simulink model "adaptive_PID"  (R2024a)
settings: Solver=FixedStepAuto  StartTime=0.0  StopTime=50  FixedStep=dt  RelTol=1e-3
undefined symbols (not defined in the file): DiscIntNeverNeededParam
libraries: simulink x1
settings Model: Creator=User  LastModifiedBy=Bocchio
settings DebuggingCC: UnconnectedInputMsg=warning  UnconnectedOutputMsg=warning  UnconnectedLineMsg=warning
settings ModelReferenceCC: EnableRefExpFcnMdlSchedulingChecks=on
settings RTWCC: GPUComputeCapability=3.5  DLArmComputeVersion=19.05

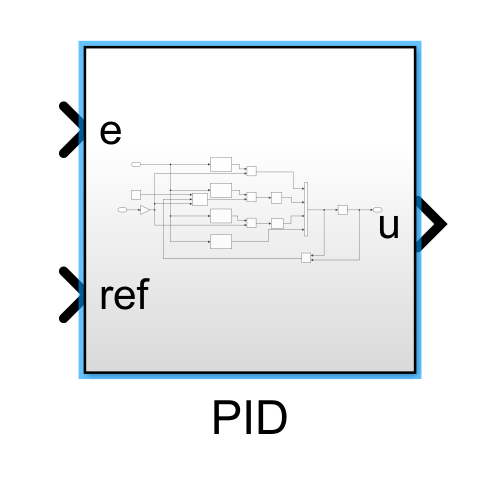
[thumbnail: Simulink's stored preview of the top-level diagram]
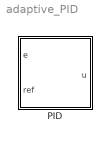
== system adaptive_PID ==
  PID : Subsystem

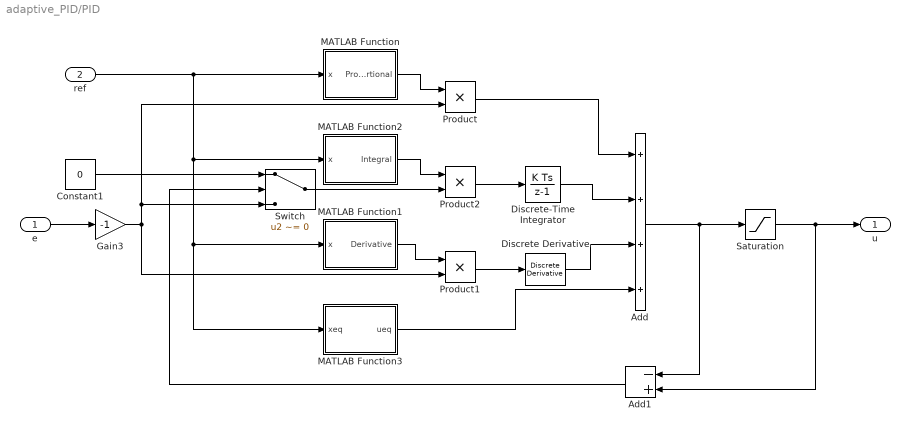
== system adaptive_PID/PID ==
  e : Inport
  ref : Inport  Port=2
  Add : Sum  Inputs=++++
  Add1 : Sum  Inputs=-+
  Constant1 : Constant  Value=0
  Discrete Derivative : simulink/Discrete/Discrete Derivative  gainval=1.0  ICPrevScaledInput=0.0  OutMin=[]  OutMax=[]  OutDataType=fixdt(1, 16)  OutScaling=2^-10  DoSatur=off
  Discrete-Time Integrator : DiscreteIntegrator  SampleTime=-1  ICPrevOutput=DiscIntNeverNeededParam  ICPrevScaledInput=DiscIntNeverNeededParam
  Gain3 : Gain  Gain=-1
  MATLAB Function : MATLAB Function  TreatAsAtomicUnit=on
  MATLAB Function1 : MATLAB Function  TreatAsAtomicUnit=on
  MATLAB Function2 : MATLAB Function  TreatAsAtomicUnit=on
  MATLAB Function3 : MATLAB Function  TreatAsAtomicUnit=on
  Product : Product
  Product1 : Product
  Product2 : Product
  Saturation : Saturate  UpperLimit=1  LowerLimit=0
  Switch : Switch  Criteria=u2 ~= 0  SaturateOnIntegerOverflow=off  InputSameDT=off
  u : Outport
  wires:
  MATLAB Function3/1(ueq) -> Add/4
  e/1 -> Gain3/1
  Saturation/1 -> u/1, Add1/2
  Add/1 -> Saturation/1, Add1/1
  Constant1/1 -> Switch/1
  Add1/1 -> Switch/2
  Gain3/1 -> Switch/3, Product/2, Product1/2
  Product/1 -> Add/1
  MATLAB Function/1(Proportional) -> Product/1
  Product1/1 -> Discrete Derivative/1
  MATLAB Function1/1(Derivative) -> Product1/1
  Product2/1 -> Discrete-Time Integrator/1
  MATLAB Function2/1(Integral) -> Product2/1
  Switch/1 -> Product2/2
  ref/1 -> MATLAB Function3/1(xeq), MATLAB Function1/1(x), MATLAB Function2/1(x), MATLAB Function/1(x)
  Discrete-Time Integrator/1 -> Add/2
  Discrete Derivative/1 -> Add/3

== matlab function adaptive_PID/PID/MATLAB Function1 ==
  data: x input; Derivative output
function Derivative = Derivative(x)

vect_pos=0.0005:0.0005:0.0185;
Kd=[-3.13284561278702	-3.15696834297852	-3.55596908354099	-4.07211547270984	-4.52885655579409	-5.03467071847558	-5.67368160958219	-6.13040622703350	-6.65900086248431	-7.20427821963870	-7.79296644491808	-8.26092294070224	-8.91573932517159	-9.51445223185005	-10.0073933096390	-10.5915963054668	-11.1707021043877	-11.7514268462752	-12.2320444397896	-12.8718043152667	-13.5079237552714	-14.0081015881516	-14.6774203594397	-15.2753544831799	-15.7810311815792	-16.5628549756766	-17.4462648456270	-18.5186925601413	-19.1642011529234	-19.8229727022934	-20.6805255599888	-21.4746229693166	-22.5687040270238	-23.8586191312697	-26.1242011711683	-28.3053228476865	-31.1934330156860];

if x<=vect_pos(1)
    Derivative=Kd(1);
elseif x>=vect_pos(1) && x<=vect_pos(end)
    Derivative=interp1(vect_pos,Kd,x);
else 
    Derivative=Kd(end);
end

== matlab function adaptive_PID/PID/MATLAB Function2 ==
  data: x input; Integral output
function Integral = Integral(x)

vect_pos=0.0005:0.0005:0.0185;
Ki=[-21.5916724653951	-21.7579270957351	-24.5078529996838	-28.0651504718742	-31.2130246688002	-34.6991121045807	-39.1031956656343	-42.2509563808898	-45.8940475657967	-49.6521166038685	-53.7093747376836	-56.9345459187291	-61.4475614470809	-65.5739100066915	-68.9712757284227	-72.9976215169708	-76.9888372609179	-80.9912108117267	-84.3036426844985	-88.7128882698608	-93.0970438571618	-96.5442855271381	-101.157251970683	-105.278233133299	-108.763373160837	-114.151727830759	-120.240216994353	-127.631423206396	-132.080289135844	-136.620563787574	-142.530845593210	-148.003790413038	-155.544232161009	-164.434368440105	-180.048832539233	-195.081193104444	-214.986141033221];

if x<=vect_pos(1)
    Integral=Ki(1);
elseif x>=vect_pos(1) && x<=vect_pos(end)
    Integral=interp1(vect_pos,Ki,x);
else 
    Integral=Ki(end);
end

== matlab function adaptive_PID/PID/MATLAB Function3 ==
  data: xeq input; ueq output
function ueq = ueq(xeq)
BallMass=0.0620;
g=9.81;
m=11.3044;
Res=4;
Kem_1=[6.72059206644115e-05	6.92145376989519e-05	6.92332150285897e-05	6.80659146785482e-05	6.99479714473845e-05	7.05722629122651e-05	6.80128124860478e-05	7.01221702001213e-05	7.05016878442255e-05	7.05515419323440e-05	6.98455307642310e-05	7.13055533313152e-05	6.96274521174565e-05	6.90147402074580e-05	6.99419931300404e-05	6.95805738707539e-05	6.93269258852514e-05	6.90843621353604e-05	7.00006512636940e-05	6.91149414076029e-05	6.97519014539535e-05	6.83573053782350e-05	6.89933518537361e-05	6.79953062557338e-05	6.77206336827605e-05	6.82595333358458e-05	6.6494e-05	6.41548968339966e-05	6.08172215535155e-05	6.05299131311581e-05	6.01818568879911e-05	5.87123846492744e-05	5.77159494392489e-05	5.52986546480238e-05	5.22809928128838e-05	4.60062308129917e-05	4.12885327629886e-05	3.57707157204477e-05	2.88156521526937e-05	2.23928764595895e-05	1.69237291476886e-05];
if xeq>=0.0185
    K1f=Kem_1(1);
    ieq = sqrt((BallMass*g)/K1f)*xeq;
    ueq = (Res*ieq)/m;
elseif xeq<0.0185 && xeq>0
    K1f = Kem_1(round(xeq*length(Kem_1)/0.02));
    ieq = sqrt((BallMass*g)/K1f)*xeq;
    ueq = (Res*ieq)/m;
else 
    K1f=Kem_1(end);
    ieq = sqrt((BallMass*g)/K1f)*xeq;
    ueq = (Res*ieq)/m;

== matlab function adaptive_PID/PID/MATLAB Function ==
  data: x input; Proportional output
function Proportional = Proportional(x)

vect_pos=0.0005:0.0005:0.0185;
Kp=[-16.4491186822817	-16.5757759456467	-18.6707436992577	-21.3807888984900	-23.7789243993465	-26.4347198714141	-29.7898695615811	-32.1879186090389	-34.9633237735508	-37.8263221689982	-40.9172508904643	-43.3742733194918	-46.8124103216076	-49.9559739936797	-52.5441788700475	-55.6115577327956	-58.6521735796689	-61.7012897448753	-64.2247897233749	-67.5838719829448	-70.9238400049996	-73.5500417245203	-77.0643240307596	-80.2037986749755	-82.8588723858806	-86.9638663649166	-91.6022416926385	-97.2330620184827	-100.622328125235	-104.081231863060	-108.583844017003	-112.753281054695	-118.497793038563	-125.270538734426	-137.166058803028	-148.618116692860	-163.782243111036];

if x<=vect_pos(1)
    Proportional=Kp(1);
elseif x>=vect_pos(1) && x<=vect_pos(end)
    Proportional=interp1(vect_pos,Kp,x);
else 
    Proportional=Kp(end);
end
